simulink model "SRV02"  (R2022b)
settings: Solver=FixedStepDiscrete  StartTime=0.0  StopTime=inf  FixedStep=0.005  RelTol=1e-3  EnableMultiTasking=on
undefined symbols (not defined in the file or in its folder): HIL, qc_get_step_size
libraries: quarc_library x4
settings Model: ExtModeTrigDuration=10000  Creator=lis3  LastModifiedBy=robert
settings SolverCC: AlgebraicLoopSolver=TrustRegion  PositivePriorityOrder=on
settings DataIOCC: ReturnWorkspaceOutputs=off
settings DebuggingCC: UnconnectedInputMsg=warning  UnconnectedOutputMsg=warning  UnconnectedLineMsg=warning  SFMachineParentedDataDiag=warning  ArithmeticOperatorsInVariantConditions=warning
settings HardwareCC: ProdBitPerPointer=32  ProdBitPerSizeT=32  ProdBitPerPtrDiffT=32  ProdLargestAtomicInteger=Long  ProdLargestAtomicFloat=Double  ProdWordSize=32  ProdHWDeviceType=ARM Compatible->ARM Cortex-A
settings ModelReferenceCC: EnableRefExpFcnMdlSchedulingChecks=on
settings SFSimCC: SimUseLocalCustomCode=off  CustomCodeUndefinedFunction=UseInterfaceOnly
settings RTWCC: Description=QUARC Linux RT ARMv7 Target (NI ELVIS III, NI myRIO) Using Toolchain  SystemTargetFile=quarc_linux_rt_armv7.tlc  TemplateMakefile=quarc_default_tmf  RTWUseLocalCustomCode=off  Toolchain=QUARC linux_rt_armv7 | gmake (64-bit Windows)  BuildConfiguration=Faster Runs  DLArmComputeVersion=19.05
settings CodeAppCC: StateflowObjectComments=on
settings STFCustomTargetCC: TargetLangStandard=C99 (ISO)  ConcurrentExecutionCompliant=on  GRTInterface=on  UseToolchainInfoCompliant=on  SystemTargetFile=quarc_linux_rt_armv7.tlc
settings GRTTargetCC: ParMdlRefBuildCompliant=off  CompOptLevelCompliant=off  CombineOutputUpdateFcns=off  MatFileLogging=off  CPPClassGenCompliant=off  GRTInterface=on  ExtMode=on  ExtModeMexFile=quarc_comm  ExtModeMexArgs='-w -d /tmp -uri %u'
settings ConfigComp: CovMetricSettings=dswe

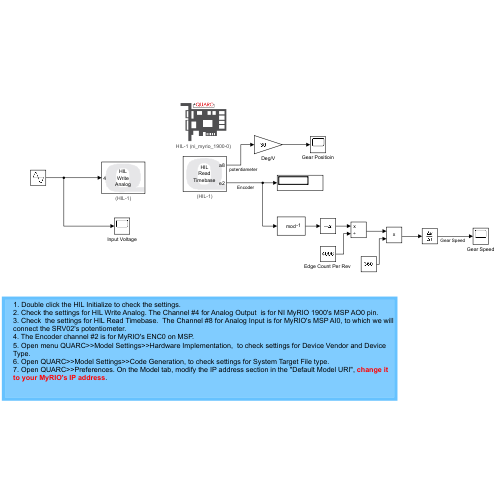
[thumbnail: Simulink's stored preview of the top-level diagram]
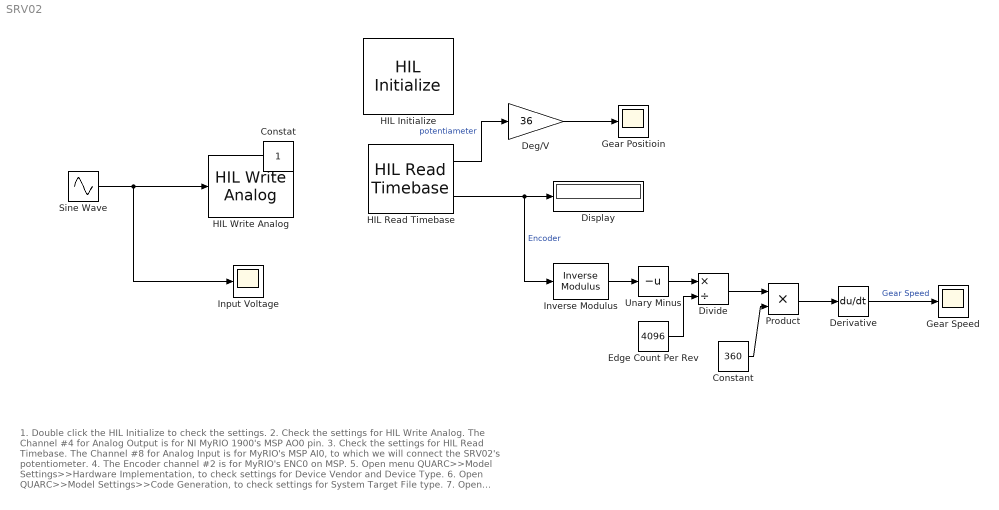
== system SRV02 ==
  note: 1. Double click the HIL Initialize to check the settings.
      | 2. Check the settings for HIL Write Analog. The Channel #4 for Analog Output is for NI MyRIO 1900's MSP AO0 pin.
      | 3. Check the settings for HIL Read Timebase. The Channel #8 for Analog Input is for MyRIO's MSP AI0, to which we will connect the SRV02's potentiometer.
      | 4. The Encoder channel #2 is for MyRIO's ENC0 on MSP.
      | 5. Open menu QUARC>>Model Settings>>Hardware Implementation, to check settings for Device Vendor and Device Type.
      | 6. Open QUARC>>Model Settings>>Code Generation, to check settings for System Target File type.
      | 7. Open QUARC>>Preferences. On the Model tab, modify the IP address section in the "Default Model URI", change it to your MyRIO's IP address .
  Constant : Constant  Value=360
  Deg/V : Gain  Gain=36
  Derivative : Derivative
  Display : Display
  Divide : Product  Inputs=*/
  "Edge Count Per Rev " : Constant  Value=4096
  Gear Positioin : Scope
  Gear Speed : Scope
  HIL Initialize : quarc_library/Data Acquisition/Generic/Configuration/HIL Initialize  object_name=HIL-1  board_type=ni_myrio_1900  board_number=0  board_options=enc0_en=1,enc1_en=1,enc2_en=1,enc3_en=1,pwm0_en=1,pwm1_en=1,pwm2_en=1,pwm3_en=1,pwm4_en=1,pwm5_en=1,pwm6_en=1,pwm7_en=1  exclusive=off  active=on  hardware_clocks=[]  clock_modes=[]  initial_clock_frequencies=[]  set_clock_params_at_start=off  set_clock_params_at_switch_in=off  set_clock_frequencies_at_start=off  set_clock_frequencies_at_switch_in=off  analog_input_channels=[0:11]  analog_input_configurations=[]  analog_input_maximums=[5 5 5 5 5 5 5 5 10 10 2.5 2.5]  analog_input_minimums=[0 0 0 0 0 0 0 0 -10 -10 -2.5 -2.5]  set_analog_input_params_at_start=off  set_analog_input_params_at_switch_in=off  analog_output_channels=[0:7]  analog_output_maximums=[5 5 5 5 10 10 2.5 2.5]  analog_output_minimums=[0 0 0 0 -10 -10 -2.5 -2.5]  initial_analog_outputs=[0]  final_analog_outputs=[0]  watchdog_analog_outputs=[]  set_analog_output_params_at_start=off  set_analog_output_params_at_switch_in=off  set_analog_outputs_at_start=on  set_analog_outputs_at_switch_in=off  set_analog_outputs_at_terminate=on  set_analog_outputs_at_switch_out=off  set_analog_outputs_on_watchdog=off  digital_input_channels=[]  digital_output_channels=[]  digital_output_configuration=[]  initial_digital_outputs=[1]  final_digital_outputs=[1]  watchdog_digital_outputs=[]  set_digital_output_params_at_start=off  set_digital_output_params_at_switch_in=off  set_digital_outputs_at_start=on  set_digital_outputs_at_switch_in=off  set_digital_outputs_at_terminate=on  set_digital_outputs_at_switch_out=off  set_digital_outputs_on_watchdog=off  encoder_channels=[2:3]  quadrature=[4]  encoder_filter_frequency=[]  initial_encoder_counts=[0]  set_encoder_params_at_start=on  set_encoder_params_at_switch_in=off  set_encoder_counts_at_start=on  set_encoder_counts_at_switch_in=off  pwm_channels=[]  pwm_modes=[0]  pwm_frequency=9765.625  pwm_configuration=[]  pwm_alignment=[]  pwm_polarity=[]  pwm_leading_deadband=[]  pwm_trailing_deadband=[]  initial_pwm_outputs=[0]  final_pwm_outputs=[0]  watchdog_pwm_outputs=[]  set_pwm_params_at_start=on  set_pwm_params_at_switch_in=off  set_pwm_outputs_at_start=on  set_pwm_outputs_at_switch_in=off  set_pwm_outputs_at_terminate=on  set_pwm_outputs_at_switch_out=off  set_pwm_outputs_on_watchdog=off  other_output_channels=[]  initial_other_outputs=[]  final_other_outputs=[]  watchdog_other_outputs=[]  set_other_outputs_at_start=off  set_other_outputs_at_switch_in=off  set_other_outputs_at_terminate=off  set_other_outputs_at_switch_out=off  set_other_outputs_on_watchdog=off
  HIL Read Timebase : quarc_library/Data Acquisition/Generic/Timebases/HIL Read Timebase  object_name=HIL-1  clock=0  analog_channels=[8]  encoder_channels=[2]  digital_channels=[]  other_channels=[]  active=on  vector_output=off  data_type_mode=Inherit via back propagation  encoder_data_type=double  digital_data_type=boolean  overflow_mode=Error on overflow  samples_in_buffer=max(ceil(1/qc_get_step_size), 1)
  HIL Write Analog : quarc_library/Data Acquisition/Generic/Immediate I//O/HIL Write Analog  object_name=HIL-1  channels=4  sample_time=-1  active=off  vector_input=off
  Input Voltage : Scope
  Inverse Modulus : quarc_library/Discontinuities/Inverse Modulus  modulus=2^32  output_derivative=off  output_revolutions=off  max_x=Inf  min_x=-Inf
  Product : Product
  Sine Wave : Sin  Amplitude=4  Frequency=3.14  SampleTime=0
  Unary Minus : UnaryMinus
  Constat : Constant  IOType=siggen
  wires:
  Sine Wave/1 -> Input Voltage/1, HIL Write Analog/1
  HIL Read Timebase/2 -> Inverse Modulus/1, Display/1  "Encoder"
  Unary Minus/1 -> Divide/1
  Inverse Modulus/1 -> Unary Minus/1
  "Edge Count Per Rev "/1 -> Divide/2
  Divide/1 -> Product/1
  Constant/1 -> Product/2
  Product/1 -> Derivative/1
  Derivative/1 -> Gear Speed/1  "Gear Speed"
  HIL Read Timebase/1 -> Deg/V/1  "potentiameter"
  Deg/V/1 -> Gear Positioin/1
